simulink model "digitaltwins_3"  (R2020b)
settings: Solver=FixedStepAuto  StartTime=0.0  StopTime=30  FixedStep=0.01  RelTol=1e-3
settings Model: Creator=skets  LastModifiedBy=PC
settings SolverCC: ConcurrentTasks=on  PositivePriorityOrder=on
settings DataIOCC: ReturnWorkspaceOutputs=off
settings OptimizationCC: BlockReduction=off  DefaultParameterBehavior=Inlined  EnhancedBackFolding=on  PassReuseOutputArgsAs=Individual arguments  ZeroExternalMemoryAtStartup=off  ZeroInternalMemoryAtStartup=off  OptimizeBlockOrder=speed  DifferentSizesBufferReuse=on  OptimizationCustomize=off  EfficientTunableParamExpr=on
settings DebuggingCC: ParameterTunabilityLossMsg=error  ArithmeticOperatorsInVariantConditions=warning
settings HardwareCC: ProdBitPerLong=64  ProdLongLongMode=on  ProdHWDeviceType=Intel->x86-64 (Linux 64)
settings SFSimCC: SimUseLocalCustomCode=off  MATLABDynamicMemAlloc=off  CustomCodeUndefinedFunction=UseInterfaceOnly
settings RTWCC: Description=Embedded Coder  SystemTargetFile=ert.tlc  GenCodeOnly=on  PackageGeneratedCodeAndArtifacts=on  PackageName=digitaltwins_3  TemplateMakefile=ert_default_tmf  RTWUseLocalCustomCode=off  Toolchain=Simulink Real-Time Toolchain  BuildConfiguration=Faster Runs  CodeExecutionProfiling=on
settings CodeAppCC: ForceParamTrailComments=on  IgnoreCustomStorageClasses=off  OperatorAnnotations=on  SimulinkDataObjDesc=on  SFDataObjDesc=on  InsertBlockDesc=on
settings ERTTargetCC: TargetLangStandard=C99 (ISO)  GenerateSampleERTMain=on  SupportContinuousTime=on  InlinedParameterPlacement=NonHierarchical  TargetOS=NativeThreadsExample  RootIOFormat=Structure reference  ERTCustomFileTemplate=example_file_process.tlc

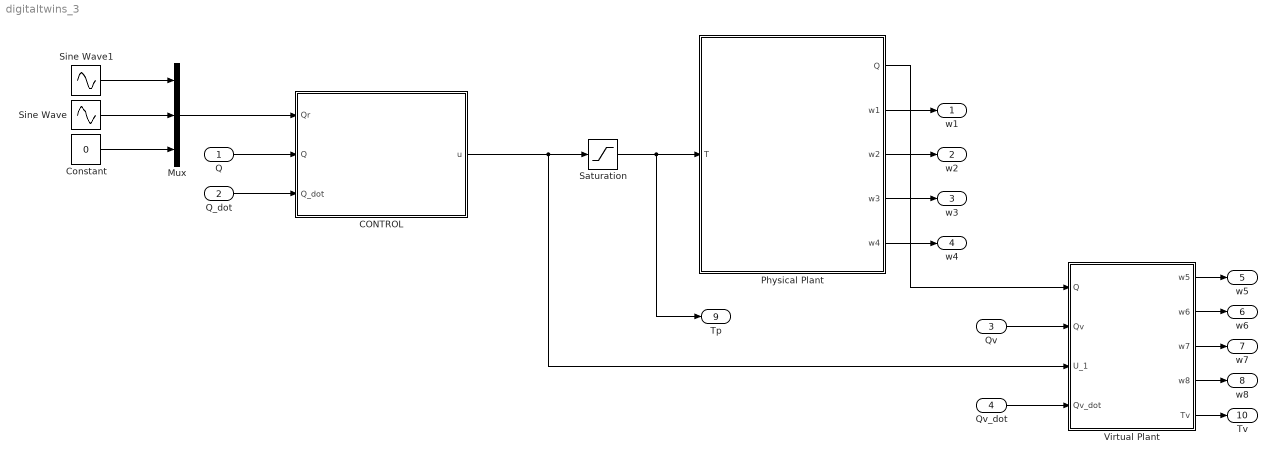
== system digitaltwins_3 ==
  Q : Inport  PortDimensions=3
  Q_dot : Inport  Port=2  PortDimensions=3
  Qv : Inport  Port=3  PortDimensions=3
  Qv_dot : Inport  Port=4  PortDimensions=3
  CONTROL : Subsystem
  Constant : Constant  Value=0
  Mux : Mux  Inputs=3
  Physical Plant : Subsystem
  Saturation : Saturate  UpperLimit=10  LowerLimit=-10
  Sine Wave : Sin  Bias=1.5  Frequency=2*pi/15  Phase=pi/2
  Sine Wave1 : Sin  Bias=1.5  Frequency=2*pi/15
  Virtual Plant : Subsystem
  w1 : Outport  VectorParamsAs1DForOutWhenUnconnected=off
  w2 : Outport  Port=2  VectorParamsAs1DForOutWhenUnconnected=off
  w3 : Outport  Port=3  VectorParamsAs1DForOutWhenUnconnected=off
  w4 : Outport  Port=4  VectorParamsAs1DForOutWhenUnconnected=off
  w5 : Outport  Port=5  VectorParamsAs1DForOutWhenUnconnected=off
  w6 : Outport  Port=6  VectorParamsAs1DForOutWhenUnconnected=off
  w7 : Outport  Port=7  VectorParamsAs1DForOutWhenUnconnected=off
  w8 : Outport  Port=8  VectorParamsAs1DForOutWhenUnconnected=off
  Tp : Outport  Port=9  PortDimensions=4  VectorParamsAs1DForOutWhenUnconnected=off
  Tv : Outport  Port=10  VectorParamsAs1DForOutWhenUnconnected=off
  wires:
  CONTROL/1(u) -> Virtual Plant/3(U_1), Saturation/1
  Physical Plant/1(Q) -> Virtual Plant/1(Q)
  Mux/1 -> CONTROL/1(Qr)
  Sine Wave1/1 -> Mux/1
  Sine Wave/1 -> Mux/2
  Constant/1 -> Mux/3
  Saturation/1 -> Tp/1, Physical Plant/1(T)
  Physical Plant/2(w1) -> w1/1
  Physical Plant/3(w2) -> w2/1
  Physical Plant/4(w3) -> w3/1
  Physical Plant/5(w4) -> w4/1
  Q/1 -> CONTROL/2(Q)
  Q_dot/1 -> CONTROL/3(Q_dot)
  Virtual Plant/1(w5) -> w5/1
  Virtual Plant/2(w6) -> w6/1
  Virtual Plant/3(w7) -> w7/1
  Virtual Plant/4(w8) -> w8/1
  Virtual Plant/5(Tv) -> Tv/1
  Qv/1 -> Virtual Plant/2(Qv)
  Qv_dot/1 -> Virtual Plant/4(Qv_dot)

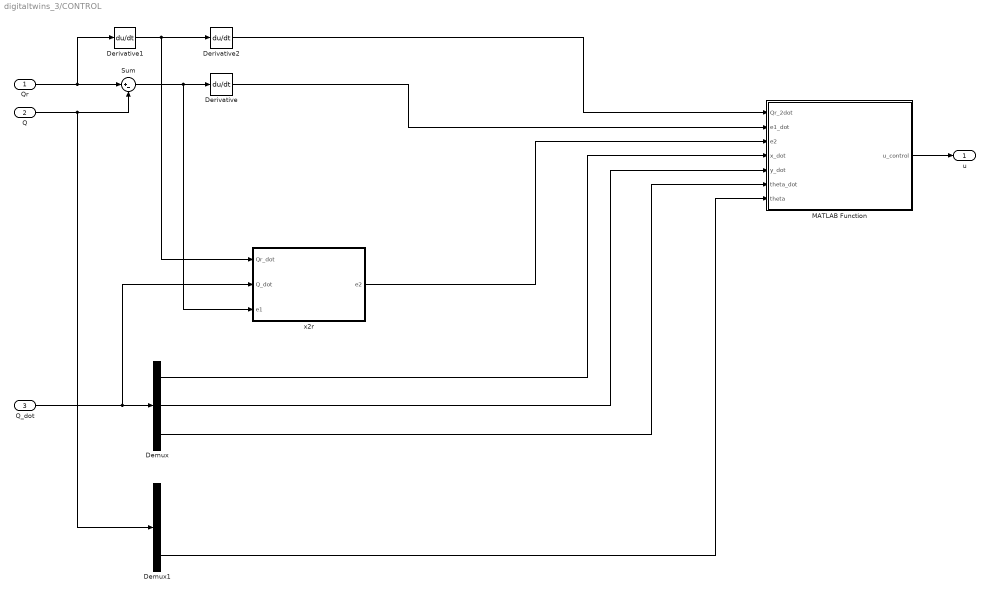
== system digitaltwins_3/CONTROL ==
  Qr : Inport
  Q : Inport  Port=2  PortDimensions=3
  Q_dot : Inport  Port=3
  Demux : Demux  Outputs=3
  Demux1 : Demux  Outputs=3
  Derivative : Derivative
  Derivative1 : Derivative
  Derivative2 : Derivative
  MATLAB Function : MATLAB Function  TreatAsAtomicUnit=on
  Sum : Sum  Inputs=|+-
  x2r : MATLAB Function  TreatAsAtomicUnit=on
  u : Outport  VectorParamsAs1DForOutWhenUnconnected=off
  wires:
  Qr/1 -> Derivative1/1, Sum/1
  Derivative1/1 -> x2r/1(Qr_dot), Derivative2/1
  MATLAB Function/1(u_control) -> u/1
  Q/1 -> Sum/2, Demux1/1
  Q_dot/1 -> x2r/2(Q_dot), Demux/1
  Demux/1 -> MATLAB Function/4(x_dot)
  Demux/2 -> MATLAB Function/5(y_dot)
  Demux/3 -> MATLAB Function/6(theta_dot)
  Demux1/3 -> MATLAB Function/7(theta)
  Sum/1 -> x2r/3(e1), Derivative/1
  Derivative2/1 -> MATLAB Function/1(Qr_2dot)
  Derivative/1 -> MATLAB Function/2(e1_dot)
  x2r/1(e2) -> MATLAB Function/3(e2)

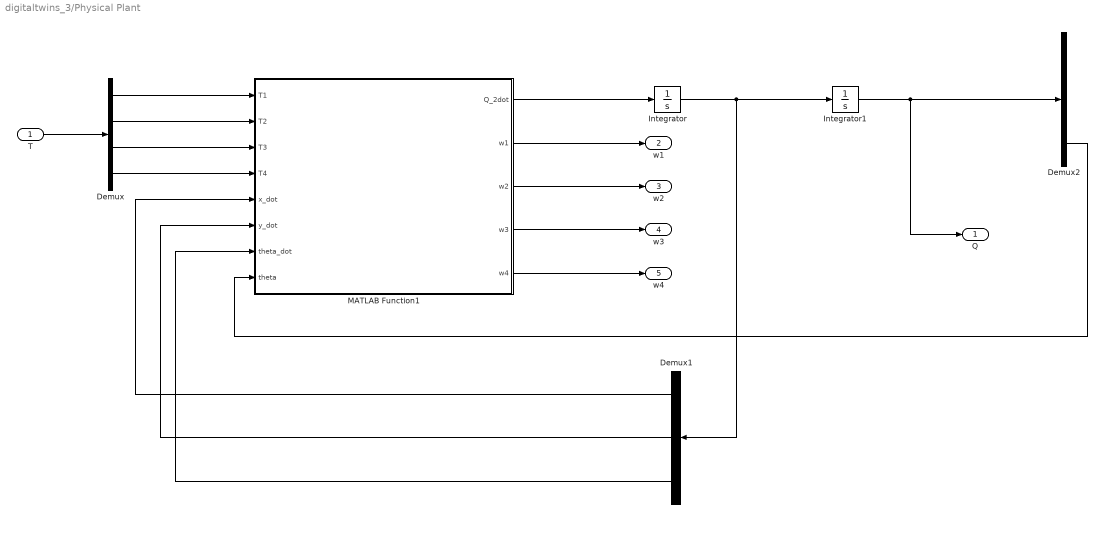
== system digitaltwins_3/Physical Plant ==
  T : Inport  PortDimensions=4
  Demux : Demux
  Demux1 : Demux  Outputs=3
  Demux2 : Demux  Outputs=3
  Integrator : Integrator
  Integrator1 : Integrator  InitialCondition=[1.5 1.5 0]
  MATLAB Function1 : MATLAB Function  TreatAsAtomicUnit=on
  Q : Outport  VectorParamsAs1DForOutWhenUnconnected=off
  w1 : Outport  Port=2  VectorParamsAs1DForOutWhenUnconnected=off
  w2 : Outport  Port=3  VectorParamsAs1DForOutWhenUnconnected=off
  w3 : Outport  Port=4  VectorParamsAs1DForOutWhenUnconnected=off
  w4 : Outport  Port=5  VectorParamsAs1DForOutWhenUnconnected=off
  wires:
  Demux/1 -> MATLAB Function1/1(T1)
  Demux/2 -> MATLAB Function1/2(T2)
  Demux/3 -> MATLAB Function1/3(T3)
  Demux/4 -> MATLAB Function1/4(T4)
  MATLAB Function1/1(Q_2dot) -> Integrator/1
  Integrator/1 -> Demux1/1, Integrator1/1
  Demux1/1 -> MATLAB Function1/5(x_dot)
  Demux1/2 -> MATLAB Function1/6(y_dot)
  Demux1/3 -> MATLAB Function1/7(theta_dot)
  Integrator1/1 -> Q/1, Demux2/1
  Demux2/3 -> MATLAB Function1/8(theta)
  T/1 -> Demux/1
  MATLAB Function1/2(w1) -> w1/1
  MATLAB Function1/3(w2) -> w2/1
  MATLAB Function1/4(w3) -> w3/1
  MATLAB Function1/5(w4) -> w4/1

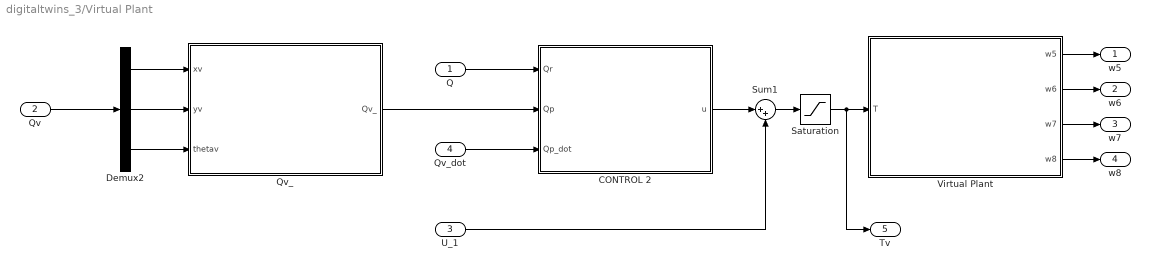
== system digitaltwins_3/Virtual Plant ==
  Q : Inport
  Qv : Inport  Port=2
  U_1 : Inport  Port=3
  Qv_dot : Inport  Port=4
  CONTROL 2 : Subsystem
  Demux2 : Demux  Outputs=3
  Qv_ : MATLAB Function  TreatAsAtomicUnit=on
  Saturation : Saturate  UpperLimit=10  LowerLimit=-10
  Sum1 : Sum  Inputs=|++
  Virtual Plant : Subsystem
  w5 : Outport  VectorParamsAs1DForOutWhenUnconnected=off
  w6 : Outport  Port=2  VectorParamsAs1DForOutWhenUnconnected=off
  w7 : Outport  Port=3  VectorParamsAs1DForOutWhenUnconnected=off
  w8 : Outport  Port=4  VectorParamsAs1DForOutWhenUnconnected=off
  Tv : Outport  Port=5  PortDimensions=4  VectorParamsAs1DForOutWhenUnconnected=off
  wires:
  Demux2/1 -> Qv_/1(xv)
  Demux2/2 -> Qv_/2(yv)
  Demux2/3 -> Qv_/3(thetav)
  Qv_/1(Qv_) -> CONTROL 2/2(Qp)
  Q/1 -> CONTROL 2/1(Qr)
  CONTROL 2/1(u) -> Sum1/1
  Sum1/1 -> Saturation/1
  U_1/1 -> Sum1/2
  Saturation/1 -> Tv/1, Virtual Plant/1(T)
  Qv/1 -> Demux2/1
  Qv_dot/1 -> CONTROL 2/3(Qp_dot)
  Virtual Plant/1(w5) -> w5/1
  Virtual Plant/2(w6) -> w6/1
  Virtual Plant/3(w7) -> w7/1
  Virtual Plant/4(w8) -> w8/1

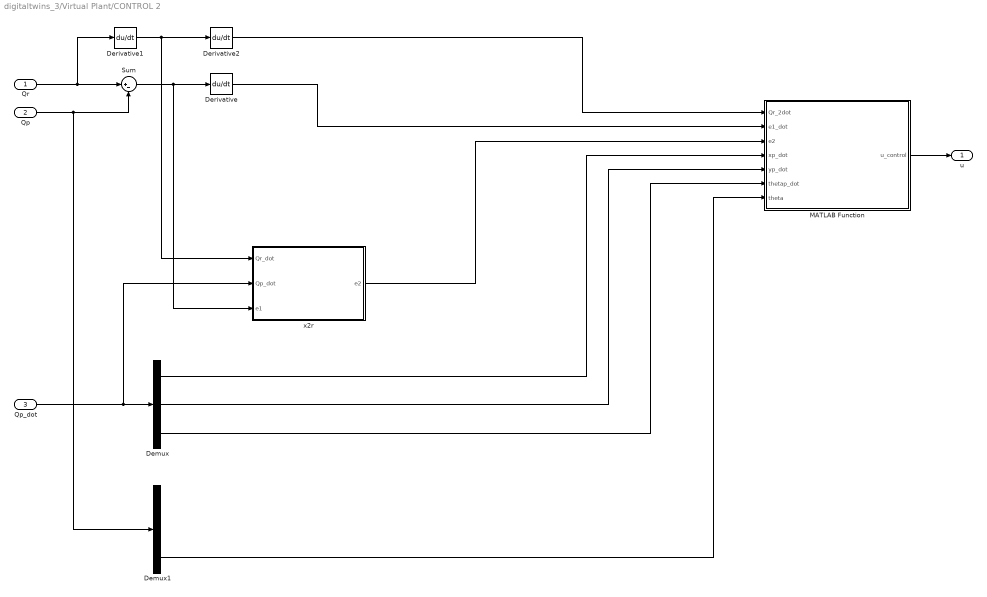
== system digitaltwins_3/Virtual Plant/CONTROL 2 ==
  Qr : Inport
  Qp : Inport  Port=2  PortDimensions=3
  Qp_dot : Inport  Port=3  PortDimensions=3
  Demux : Demux  Outputs=3
  Demux1 : Demux  Outputs=3
  Derivative : Derivative
  Derivative1 : Derivative
  Derivative2 : Derivative
  MATLAB Function : MATLAB Function  TreatAsAtomicUnit=on
  Sum : Sum  Inputs=|+-
  x2r : MATLAB Function  TreatAsAtomicUnit=on
  u : Outport  VectorParamsAs1DForOutWhenUnconnected=off
  wires:
  Qr/1 -> Derivative1/1, Sum/1
  Derivative1/1 -> x2r/1(Qr_dot), Derivative2/1
  MATLAB Function/1(u_control) -> u/1
  Qp/1 -> Sum/2, Demux1/1
  Qp_dot/1 -> x2r/2(Qp_dot), Demux/1
  Demux/1 -> MATLAB Function/4(xp_dot)
  Demux/2 -> MATLAB Function/5(yp_dot)
  Demux/3 -> MATLAB Function/6(thetap_dot)
  Demux1/3 -> MATLAB Function/7(theta)
  Sum/1 -> x2r/3(e1), Derivative/1
  x2r/1(e2) -> MATLAB Function/3(e2)
  Derivative2/1 -> MATLAB Function/1(Qr_2dot)
  Derivative/1 -> MATLAB Function/2(e1_dot)

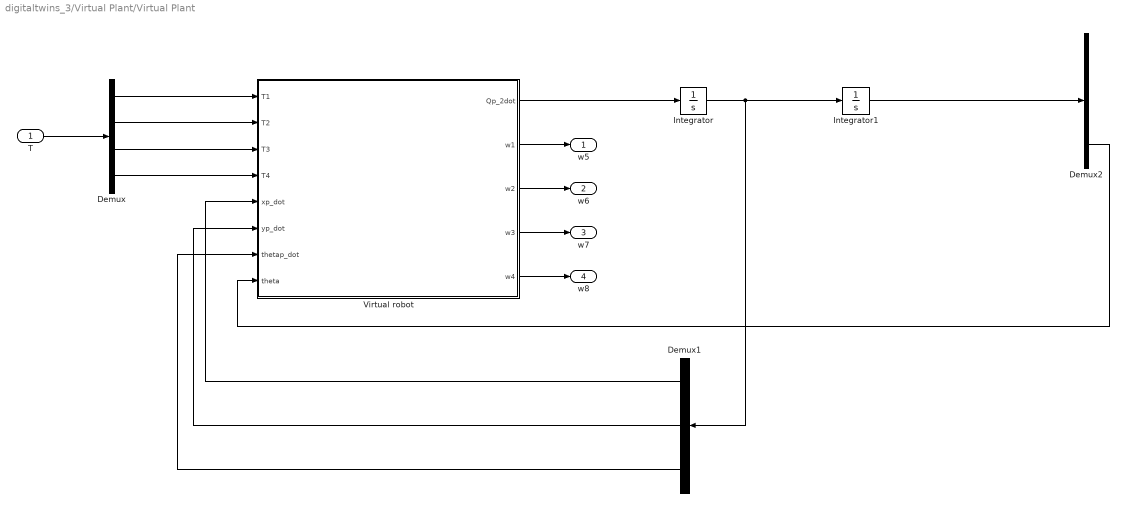
== system digitaltwins_3/Virtual Plant/Virtual Plant ==
  T : Inport  PortDimensions=4
  Demux : Demux
  Demux1 : Demux  Outputs=3
  Demux2 : Demux  Outputs=3
  Integrator : Integrator
  Integrator1 : Integrator  InitialCondition=[1.5 1.5 0]
  Virtual robot : MATLAB Function  TreatAsAtomicUnit=on
  w5 : Outport  VectorParamsAs1DForOutWhenUnconnected=off
  w6 : Outport  Port=2  VectorParamsAs1DForOutWhenUnconnected=off
  w7 : Outport  Port=3  VectorParamsAs1DForOutWhenUnconnected=off
  w8 : Outport  Port=4  VectorParamsAs1DForOutWhenUnconnected=off
  wires:
  Demux/1 -> Virtual robot/1(T1)
  Demux/2 -> Virtual robot/2(T2)
  Demux/3 -> Virtual robot/3(T3)
  Demux/4 -> Virtual robot/4(T4)
  Virtual robot/1(Qp_2dot) -> Integrator/1
  Integrator/1 -> Demux1/1, Integrator1/1
  Demux1/1 -> Virtual robot/5(xp_dot)
  Demux1/2 -> Virtual robot/6(yp_dot)
  Demux1/3 -> Virtual robot/7(thetap_dot)
  Integrator1/1 -> Demux2/1
  Demux2/3 -> Virtual robot/8(theta)
  T/1 -> Demux/1
  Virtual robot/2(w1) -> w5/1
  Virtual robot/3(w2) -> w6/1
  Virtual robot/4(w3) -> w7/1
  Virtual robot/5(w4) -> w8/1

== matlab function digitaltwins_3/Virtual Plant/CONTROL 2/x2r ==
  data: Qr_dot input; Qp_dot input; e2 output; e1 input
function e2  = fcn(Qr_dot,Qp_dot,e1)

k1 = [10 0 0;
      0 10 0;
      0 0 10];
 
%x2r_dot = (Qr_2dot+k1*e1_dot);
x2r = Qr_dot + k1*e1;
e2 = x2r - Qp_dot;

== matlab function digitaltwins_3/Physical Plant/MATLAB Function1 ==
  data: T1 input; Q_2dot output; T2 input; T3 input; T4 input; x_dot input; y_dot input; theta_dot input; theta input; w1 output; w2 output; w3 output; w4 output
function [Q_2dot,w1,w2,w3,w4] = fcn(T1, T2, T3, T4,x_dot,y_dot,theta_dot,theta)
m=5;
I=5;
Ib=0.1;
l1= 0.3;
l2=0.3;
r=0.097/2;
g=9.81;
u=0.01;
N = m*g/4;
M=[(m+4*Ib/(r*r)) 0 0; 0 (m+4*Ib/(r*r)) 0; 0 0 (I+4*Ib*(l1+l2)*(l1+l2)/(r*r))];
C= [(m+4*Ib/(r*r))*y_dot*theta_dot;-(m+4*Ib/(r*r))*x_dot*theta_dot;0 ];
B=(1/r)*[(cos(theta)+sin(theta)) (cos(theta)-sin(theta)) (cos(theta)+sin(theta)) (cos(theta)-sin(theta));
         (-cos(theta)+sin(theta)) (cos(theta)+sin(theta)) (-cos(theta)+sin(theta)) (cos(theta)+sin(theta)); 
         (-(l1+l2)) (l1+l2) (l1+l2) (-(l1+l2)) ];
T=[T1;T2;T3;T4];
xm= cos(theta)*x_dot+sin(theta)*y_dot;
ym= -sin(theta)*x_dot+cos(theta)*y_dot;
w1 = (1/r)*(xm-ym-(l1+l2)*theta_dot);
w2 = (1/r)*(xm+ym+(l1+l2)*theta_dot);
w3 = (1/r)*(xm-ym+(l1+l2)*theta_dot);
w4 = (1/r)*(xm+ym-(l1+l2)*theta_dot);
w_max = 2*pi;
if w1 > w_max
    w1 = w_max;
elseif w1 < -w_max
    w1 = -w_max;
end
if w2 > w_max
    w2 = w_max;
elseif w2 < -w_max
    w2 = -w_max;
end
if w3 > w_max
    w3 = w_max;
elseif w3 < -w_max
    w3 = -w_max;
end
if w4 > w_max
    w4 = w_max;
elseif w4 < -w_max
    w4 = -w_max;
end
Xi=[u*r*N*sign(w1);u*r*N*sign(w2);u*r*N*sign(w3);u*N*r*sign(w4)];

Q_2dot=inv(M)*(B*T-C-B*Xi);

== matlab function digitaltwins_3/CONTROL/MATLAB Function ==
  data: Qr_2dot input; u_control output; e1_dot input; e2 input; x_dot input; y_dot input; theta_dot input; theta input
function u_control = fcn(Qr_2dot,e1_dot,e2,x_dot,y_dot,theta_dot,theta)

m=5;
I=5;
Ib=0.1;
l1= 0.3;
l2=0.3;
r=0.097/2;
g=9.81;
u=0.01;
N = m*g/4;
M=[(m+4*Ib/(r*r)) 0 0; 0 (m+4*Ib/(r*r)) 0; 0 0 (I+4*Ib*(l1+l2)*(l1+l2)/(r*r))];
C= [(m+4*Ib/(r*r))*y_dot*theta_dot;-(m+4*Ib/(r*r))*x_dot*theta_dot;0 ];
B=(1/r)*[(cos(theta)+sin(theta)) (cos(theta)-sin(theta)) (cos(theta)+sin(theta)) (cos(theta)-sin(theta));
    (-cos(theta)+sin(theta)) (cos(theta)+sin(theta)) (-cos(theta)+sin(theta)) (cos(theta)+sin(theta)); 
    (-(l1+l2)) (l1+l2) (l1+l2) (-(l1+l2)) ];

xm= cos(theta)*x_dot+sin(theta)*y_dot;
ym= -sin(theta)*x_dot+cos(theta)*y_dot;
w1 = (1/r)*(xm-ym-(l1+l2)*theta_dot);
w2 = (1/r)*(xm+ym+(l1+l2)*theta_dot);
w3 = (1/r)*(xm-ym+(l1+l2)*theta_dot);
w4 = (1/r)*(xm+ym-(l1+l2)*theta_dot);
w_max = 2*pi;
if w1 > w_max
    w1 = w_max;
elseif w1 < -w_max
    w1 = -w_max;
end
if w2 > w_max
    w2 = w_max;
elseif w2 < -w_max
    w2 = -w_max;
end
if w3 > w_max
    w3 = w_max;
elseif w3 < -w_max
    w3 = -w_max;
end
if w4 > w_max
    w4 = w_max;
elseif w4 < -w_max
    w4 = -w_max;
end
Xi=[u*r*N*sign(w1);u*r*N*sign(w2);u*r*N*sign(w3);u*N*r*sign(w4)];

k1 = [4 0 0;
      0 4 0;
      0 0 4];
k2 = [4 0 0;
      0 4 0;
      0 0 4];
  
u_control = B'*inv(B*B')*M*((Qr_2dot+k1*e1_dot)+inv(M)*C+inv(M)*B*Xi+k2*e2);

== matlab function digitaltwins_3/CONTROL/x2r ==
  data: Qr_dot input; Q_dot input; e2 output; e1 input
function e2  = fcn(Qr_dot,Q_dot,e1)

k1 = [4 0 0;
      0 4 0;
      0 0 4];
 
%x2r_dot = (Qr_2dot+k1*e1_dot);
x2r = Qr_dot + k1*e1;
e2 = x2r - Q_dot;

== matlab function digitaltwins_3/Virtual Plant/Qv_ ==
  data: Qv_ output; xv input; yv input; thetav input
function Qv_ = fcn(xv, yv,thetav)

xp_t0 = 1.5;
yp_t0 = 1.5;
thetap_t0 = 0;
xv_t0 = 1.5;
yv_t0 = 1.5;
thetav_t0 = 0;
delta_theta = thetap_t0 - thetav_t0;
delta_x = xp_t0 - xv_t0*cos(delta_theta) - yv_t0*sin(delta_theta);
delta_y = yp_t0 - xv_t0*sin(delta_theta) - yv_t0*cos(delta_theta);

T_delta = [ 1 0 0 delta_x;
            0 1 0 delta_y;
            0 0 1 delta_theta;
            0 0 0 1];
R_delta = [ cos(delta_theta) -sin(delta_theta) 0 0;
            sin(delta_theta) cos(delta_theta) 0 0;
            0 0 1 0;
            0 0 0 1 ];   
H = T_delta*R_delta;
Qv_temp = H*[ xv; yv; thetav; 1];
Qv_ = [Qv_temp(1);Qv_temp(2);Qv_temp(3)];

== matlab function digitaltwins_3/Virtual Plant/Virtual Plant/Virtual robot ==
  data: T1 input; Qp_2dot output; T2 input; T3 input; T4 input; xp_dot input; yp_dot input; thetap_dot input; theta input; w1 output; w2 output; w3 output; w4 output
function [Qp_2dot,w1,w2,w3,w4]  = fcn(T1, T2, T3, T4,xp_dot,yp_dot,thetap_dot,theta)
m=5;
I=5;
Ib=0.1;
l1= 0.3;
l2=0.3;
r=0.097/2;
g=9.81;
u=0.01;
N = m*g/4;
M=[(m+4*Ib/(r*r)) 0 0; 0 (m+4*Ib/(r*r)) 0; 0 0 (I+4*Ib*(l1+l2)*(l1+l2)/(r*r))];
C= [(m+4*Ib/(r*r))*yp_dot*thetap_dot;-(m+4*Ib/(r*r))*xp_dot*thetap_dot;0 ];
B=(1/r)*[(cos(theta)+sin(theta)) (cos(theta)-sin(theta)) (cos(theta)+sin(theta)) (cos(theta)-sin(theta));
         (-cos(theta)+sin(theta)) (cos(theta)+sin(theta)) (-cos(theta)+sin(theta)) (cos(theta)+sin(theta)); 
         (-(l1+l2)) (l1+l2) (l1+l2) (-(l1+l2)) ];
T=[T1;T2;T3;T4];
xm= cos(theta)*xp_dot+sin(theta)*yp_dot;
ym= -sin(theta)*xp_dot+cos(theta)*yp_dot;
w1 = (1/r)*(xm-ym-(l1+l2)*thetap_dot);
w2 = (1/r)*(xm+ym+(l1+l2)*thetap_dot);
w3 = (1/r)*(xm-ym+(l1+l2)*thetap_dot);
w4 = (1/r)*(xm+ym-(l1+l2)*thetap_dot);
w_max = 2*pi;
if w1 > w_max
    w1 = w_max;
elseif w1 < -w_max
    w1 = -w_max;
end
if w2 > w_max
    w2 = w_max;
elseif w2 < -w_max
    w2 = -w_max;
end
if w3 > w_max
    w3 = w_max;
elseif w3 < -w_max
    w3 = -w_max;
end
if w4 > w_max
    w4 = w_max;
elseif w4 < -w_max
    w4 = -w_max;
end
Xi=[u*r*N*sign(w1);u*r*N*sign(w2);u*r*N*sign(w3);u*N*r*sign(w4)];

Qp_2dot=inv(M)*(B*T-C-B*Xi);

== matlab function digitaltwins_3/Virtual Plant/CONTROL 2/MATLAB Function ==
  data: Qr_2dot input; u_control output; e1_dot input; e2 input; xp_dot input; yp_dot input; thetap_dot input; theta input
function u_control = fcn(Qr_2dot,e1_dot,e2,xp_dot,yp_dot,thetap_dot,theta)

m=5;
I=5;
Ib=0.1;
l1= 0.3;
l2=0.3;
r=0.097/2;
g=9.81;
u=0.01;
N = m*g/4;
M=[(m+4*Ib/(r*r)) 0 0; 0 (m+4*Ib/(r*r)) 0; 0 0 (I+4*Ib*(l1+l2)*(l1+l2)/(r*r))];
C= [(m+4*Ib/(r*r))*yp_dot*thetap_dot;-(m+4*Ib/(r*r))*xp_dot*thetap_dot;0 ];
B=(1/r)*[(cos(theta)+sin(theta)) (cos(theta)-sin(theta)) (cos(theta)+sin(theta)) (cos(theta)-sin(theta));
    (-cos(theta)+sin(theta)) (cos(theta)+sin(theta)) (-cos(theta)+sin(theta)) (cos(theta)+sin(theta)); 
    (-(l1+l2)) (l1+l2) (l1+l2) (-(l1+l2)) ];

xm= cos(theta)*xp_dot+sin(theta)*yp_dot;
ym= -sin(theta)*xp_dot+cos(theta)*yp_dot;
w1 = (1/r)*(xm-ym-(l1+l2)*thetap_dot);
w2 = (1/r)*(xm+ym+(l1+l2)*thetap_dot);
w3 = (1/r)*(xm-ym+(l1+l2)*thetap_dot);
w4 = (1/r)*(xm+ym-(l1+l2)*thetap_dot);
w_max = 2*pi;
if w1 > w_max
    w1 = w_max;
elseif w1 < -w_max
    w1 = -w_max;
end
if w2 > w_max
    w2 = w_max;
elseif w2 < -w_max
    w2 = -w_max;
end
if w3 > w_max
    w3 = w_max;
elseif w3 < -w_max
    w3 = -w_max;
end
if w4 > w_max
    w4 = w_max;
elseif w4 < -w_max
    w4 = -w_max;
end
Xi=[u*r*N*sign(w1);u*r*N*sign(w2);u*r*N*sign(w3);u*N*r*sign(w4)];

k1 = [10 0 0;
      0 10 0;
      0 0 10];
k2 = [10 0 0;
      0 10 0;
      0 0 10];
  
u_control = B'*inv(B*B')*M*((Qr_2dot+k1*e1_dot)+inv(M)*C+inv(M)*B*Xi+k2*e2);
